simulink model "kinematic_bicycle"  (R2017b)
settings: Solver=FixedStepAuto  StartTime=0.0  StopTime=5  FixedStep=0.002  RelTol=1e-3
values from neighbouring files (symbols this model uses):
  input_type = 3    [main_bicycle.m]    (also in main_differential_steer.m; main_dynamic_bicycle.m)
  l_f = 1.07    [main_bicycle.m]
  l_r = 0.936    [main_bicycle.m]
  psi_init = 0    [main_bicycle.m]
  v_const = 1    [main_bicycle.m]    (also in main_dynamic_bicycle.m = 0.9)
  x_init = 0    [main_bicycle.m]
  y_init = 0    [main_bicycle.m]
settings Model: Creator=zhenghe3  LastModifiedBy=zhenghe3

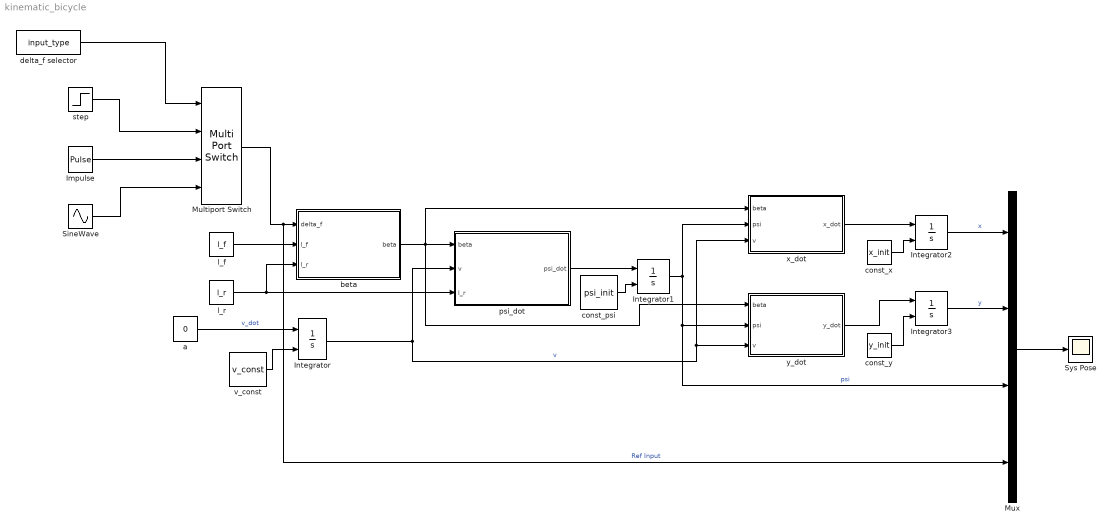
== system kinematic_bicycle ==
  Impulse : DiscretePulseGenerator  PulseType=Time based  Period=1  PulseWidth=50
  Integrator{,1..3} (4 alike) : Integrator  InitialConditionSource=external
  Multiport Switch : MultiPortSwitch
  Mux : Mux
  SineWave : Sin  Frequency=5  SampleTime=0
  Sys Pose : Scope
  a : Constant  Value=0
  beta : MATLAB Function  TreatAsAtomicUnit=on
  const_psi : Constant  Value=psi_init
  const_x : Constant  Value=x_init
  const_y : Constant  Value=y_init
  delta_f selector : Constant  Value=input_type
  l_f : Constant  Value=l_f
  l_r : Constant  Value=l_r
  psi_dot : MATLAB Function  TreatAsAtomicUnit=on
  step : Step  Time=0  SampleTime=0
  v_const : Constant  Value=v_const
  x_dot : MATLAB Function  TreatAsAtomicUnit=on
  y_dot : MATLAB Function  TreatAsAtomicUnit=on
  wires:
  a/1 -> Integrator/1  "v_dot"
  Integrator/1 -> x_dot/3(v), y_dot/3(v), psi_dot/2(v)  "v"
  beta/1(beta) -> y_dot/1(beta), psi_dot/1(beta), x_dot/1(beta)
  psi_dot/1(psi_dot) -> Integrator1/1
  Integrator1/1 -> Mux/3, y_dot/2(psi), x_dot/2(psi)  "psi"
  y_dot/1(y_dot) -> Integrator3/1
  x_dot/1(x_dot) -> Integrator2/1
  Integrator2/1 -> Mux/1  "x"
  Integrator3/1 -> Mux/2  "y"
  Mux/1 -> Sys Pose/1
  v_const/1 -> Integrator/2
  const_x/1 -> Integrator2/2
  const_y/1 -> Integrator3/2
  const_psi/1 -> Integrator1/2
  Multiport Switch/1 -> Mux/4, beta/1(delta_f)  "Ref Input"
  delta_f selector/1 -> Multiport Switch/1
  step/1 -> Multiport Switch/2
  Impulse/1 -> Multiport Switch/3
  SineWave/1 -> Multiport Switch/4
  l_f/1 -> beta/2(l_f)
  l_r/1 -> psi_dot/3(l_r), beta/3(l_r)

== matlab function kinematic_bicycle/y_dot ==
  data: beta input; y_dot output; psi input; v input
function y_dot = calc_y_dot(beta, psi, v)

y_dot = v * sin(psi + beta);

== matlab function kinematic_bicycle/beta ==
  data: delta_f input; beta output; l_f input; l_r input
function beta = calc_beta(delta_f, l_f, l_r)

beta = atan(l_f/(l_f+l_r) * tan(delta_f));

== matlab function kinematic_bicycle/x_dot ==
  data: beta input; x_dot output; psi input; v input
function x_dot = calc_x_dot(beta, psi, v)

x_dot = v * cos(psi + beta);

== matlab function kinematic_bicycle/psi_dot ==
  data: beta input; psi_dot output; v input; l_r input
function psi_dot = calc_psi_dot(beta, v, l_r)

psi_dot = v / l_r * sin(beta);
